simulink model "MPC_linear_2015"  (R2015a)
settings: Solver=ode45  StartTime=0.0  StopTime=10.0  RelTol=1e-3
values from neighbouring files (symbols this model uses):
  AINEQ = mpcobj.AINEQ    [teste.m]
  cmd_lb = -1e5    (= -100000)    [initParams.m]    (also in teste.m = -2000)
  cmd_ub = 1e5    (= 100000)    [initParams.m]    (also in teste.m = 2000)
  dA = d_sys.a    [teste.m]
  dB = d_sys.b    [teste.m]
  dC = d_sys.c    [teste.m]
  dD = d_sys.d    [teste.m]
  F1 = mpcobj.F1    [teste.m]
  F2 = mpcobj.F2    [teste.m]
  F3 = mpcobj.F3    [teste.m]
  G1 = mpcobj.G1    [teste.m]
  G2 = mpcobj.G2    [teste.m]
  G3 = mpcobj.G3    [teste.m]
  G4 = mpcobj.G4    [teste.m]
  H = mpcobj.H    [teste.m]
  lb = [ -pi/36; -pi; -pi; -pi/36 ]    [initParams.m]    (also in teste.m = -0.0872664625997)
  openloop = 0    [teste.m]
  PI = mpcobj.PI_E    [teste.m]
  rate_factor = 14    [teste.m]
  rate_lb = -rate_ub    (= -1.3962634016e-05)    [teste.m]
  rate_th = pi*Ts/180    (= 1.3962634016e-06)    [teste.m]
  rate_ub = 10*pi*Ts/180    (= 1.3962634016e-05)    [teste.m]
  ub = -lb    [initParams.m]    (also in teste.m = 0.0872664625997)
settings Model: Creator=zoero  LastModifiedBy=zoero

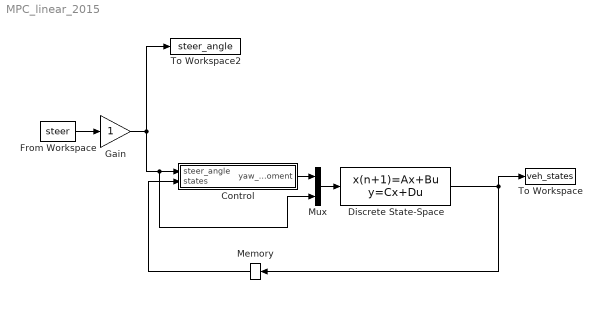
== system MPC_linear_2015 ==
  "Control " : Subsystem  TreatAsAtomicUnit=on
  Discrete State-Space : DiscreteStateSpace  A=dA  B=dB  C=dC  D=dD  X0=[0 0 0 0]  SampleTime=8e-5
  From Workspace : FromWorkspace  VariableName=steer  SampleTime=0
  Gain : Gain
  Memory : Memory  X0=[0,0,0,0]
  Mux : Mux  Inputs=2
  To Workspace : ToWorkspace  VariableName=veh_states  SaveFormat=Timeseries  SampleTime=-1
  To Workspace2 : ToWorkspace  VariableName=steer_angle  SaveFormat=Timeseries  SampleTime=-1
  wires:
  From Workspace/1 -> Gain/1
  Gain/1 -> To Workspace2/1, Mux/2, "Control "/1(steer_angle)
  Memory/1 -> "Control "/2(states)
  Discrete State-Space/1 -> To Workspace/1, Memory/1
  "Control "/1(yaw_moment) -> Mux/1
  Mux/1 -> Discrete State-Space/1

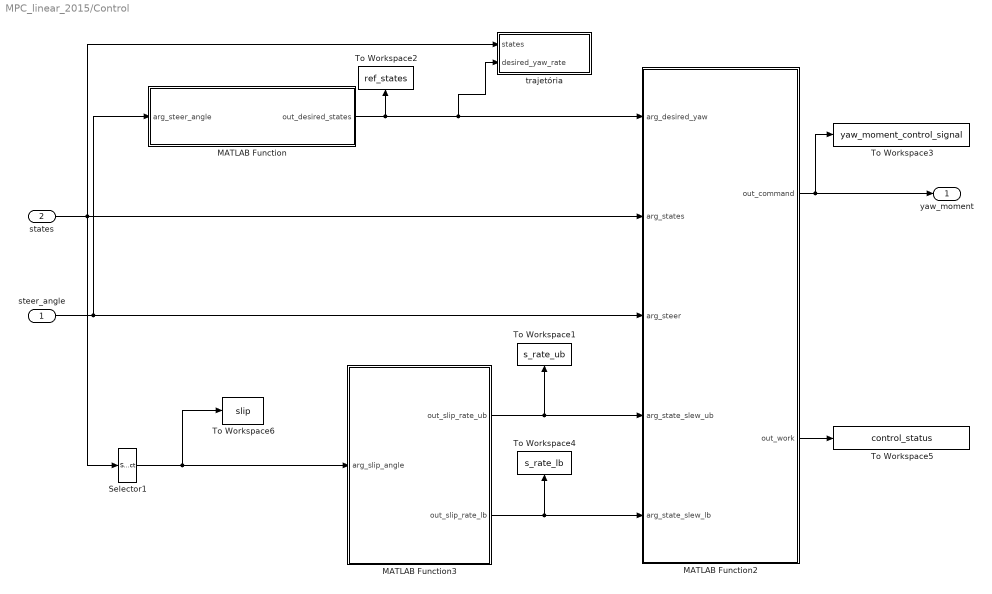
== system MPC_linear_2015/Control  ==
  steer_angle : Inport
  states : Inport  Port=2
  MATLAB Function : MATLAB Function  TreatAsAtomicUnit=on
  MATLAB Function2 : MATLAB Function  TreatAsAtomicUnit=on  SystemSampleTime=8e-5
  MATLAB Function3 : MATLAB Function  TreatAsAtomicUnit=on
  Selector1 : Selector  InputPortWidth=4  Indices=[1]
  To Workspace1 : ToWorkspace  VariableName=s_rate_ub  SaveFormat=Timeseries  SampleTime=-1
      settings: MaxDataPoints=Inf
  To Workspace2 : ToWorkspace  VariableName=ref_states  SaveFormat=Timeseries  SampleTime=-1
      settings: MaxDataPoints=Inf
  To Workspace3 : ToWorkspace  VariableName=yaw_moment_control_signal  SaveFormat=Timeseries  SampleTime=-1
      settings: MaxDataPoints=Inf
  To Workspace4 : ToWorkspace  VariableName=s_rate_lb  SaveFormat=Timeseries  SampleTime=-1
      settings: MaxDataPoints=Inf
  To Workspace5 : ToWorkspace  VariableName=control_status  SaveFormat=Timeseries  SampleTime=-1
      settings: MaxDataPoints=Inf
  To Workspace6 : ToWorkspace  VariableName=slip  SaveFormat=Timeseries  SampleTime=-1
      settings: MaxDataPoints=Inf
  trajetória : Subsystem
  yaw_moment : Outport
  wires:
  MATLAB Function2/1(out_command) -> To Workspace3/1, yaw_moment/1
  steer_angle/1 -> MATLAB Function/1(arg_steer_angle), MATLAB Function2/3(arg_steer)
  MATLAB Function3/1(out_slip_rate_ub) -> To Workspace1/1, MATLAB Function2/4(arg_state_slew_ub)
  MATLAB Function3/2(out_slip_rate_lb) -> MATLAB Function2/5(arg_state_slew_lb), To Workspace4/1
  states/1 -> MATLAB Function2/2(arg_states), Selector1/1, trajetória/1(states)
  MATLAB Function2/2(out_work) -> To Workspace5/1
  Selector1/1 -> To Workspace6/1, MATLAB Function3/1(arg_slip_angle)
  MATLAB Function/1(out_desired_states) -> To Workspace2/1, trajetória/2(desired_yaw_rate), MATLAB Function2/1(arg_desired_yaw)

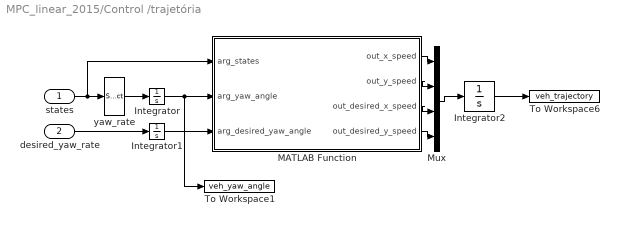
== system MPC_linear_2015/Control /trajetória ==
  states : Inport
  desired_yaw_rate : Inport  Port=2
  Integrator : Integrator
  Integrator1 : Integrator
  Integrator2 : Integrator
  MATLAB Function : MATLAB Function  TreatAsAtomicUnit=on
  Mux : Mux
  To Workspace1 : ToWorkspace  VariableName=veh_yaw_angle  SaveFormat=Timeseries  SampleTime=-1
  To Workspace6 : ToWorkspace  VariableName=veh_trajectory  SaveFormat=Timeseries  SampleTime=-1
  yaw_rate : Selector  InputPortWidth=4  Indices=[2]
  wires:
  states/1 -> yaw_rate/1, MATLAB Function/1(arg_states)
  yaw_rate/1 -> Integrator/1
  Integrator/1 -> To Workspace1/1, MATLAB Function/2(arg_yaw_angle)
  Integrator1/1 -> MATLAB Function/3(arg_desired_yaw_angle)
  desired_yaw_rate/1 -> Integrator1/1
  MATLAB Function/1(out_x_speed) -> Mux/1
  MATLAB Function/2(out_y_speed) -> Mux/2
  MATLAB Function/3(out_desired_x_speed) -> Mux/3
  MATLAB Function/4(out_desired_y_speed) -> Mux/4
  Mux/1 -> Integrator2/1
  Integrator2/1 -> To Workspace6/1

== matlab function MPC_linear_2015/Control /MATLAB Function ==
  data: arg_steer_angle input; out_desired_states output; uspeed parameter
function out_desired_states  = desired_states(arg_steer_angle,  uspeed)

persistent mu_g;
persistent Ku;
persistent l;

if isempty(Ku)
    modelParams = coder.load( 'modelParam.mat' );
    mu_g = modelParams.friction_coefficient*modelParams.g;
    l = modelParams.l;
    Ku = modelParams.Ku;
end

aux = (l + Ku*uspeed*uspeed);
desired_yaw_rate = uspeed*arg_steer_angle/aux;


desired_yaw_rate = min([abs(desired_yaw_rate), abs(mu_g/uspeed)])*sign(arg_steer_angle);


out_desired_states = desired_yaw_rate;

end

== matlab function MPC_linear_2015/Control /MATLAB Function2 ==
  data: arg_desired_yaw input; out_command output size=1; arg_states input; arg_steer input; arg_state_slew_ub input; arg_state_slew_lb input; G1 parameter; G2 parameter; G3 parameter; G4 parameter; F1 parameter; F2 parameter; F3 parameter; cmd_lb parameter; cmd_ub parameter; H parameter; AINEQ parameter; PI parameter; ub parameter; lb parameter; out_work output; openloop parameter
function [out_command, out_work]= mpc(arg_desired_yaw, arg_states, arg_steer, ...
arg_state_slew_ub, arg_state_slew_lb, G1, G2, G3, G4, F1, F2, F3, cmd_lb,...
cmd_ub, H, AINEQ, PI, ub,lb, openloop)
 persistent U
 persistent QP
 persistent N
 persistent np
 persistent nc
 persistent nu
% persistent on
 if isempty(U)
     U = 0;
     N = 101;
     np = 4;
     nc = 1;
     nu = 2;
 %    on = 0;
 end
 
 if  openloop ~= 0
    out_command = 0;
    out_work = 0;
    return
 end
  %if on == 0
  %  if ( abs(arg_desired_yaw) > pi/180) || ( abs(arg_states(1)) > 4*pi/180 )
  %      on = 1;
  %  else
  %      out_command = 0;
  %      return;
  %  end
  %else
  %  if ( abs(arg_desired_yaw) < pi/180 ) && ( abs(arg_states(1)) < 4*pi/180 )
  %      out_command = 0;
  %      %on = 0;
  %      %return;
  %  end
  %end
 
 TRACK = arg_desired_yaw*ones(N,1);
 TRACK = reshape(TRACK,[],1);
 G5 = zeros(8*N,1);
 G5( 6*N+1:7*N, : ) = repmat(arg_state_slew_ub,N,1);
 G5( 7*N+1:8*N, : ) = -repmat(arg_state_slew_lb,N,1);
 
 B_INEQ = ( G1 + G4 )*arg_states + G2*U + G3 + G5;
 F = F1*arg_states + F2*TRACK + F3*[0; arg_steer];
 F = PI'*F;
 aux_cmd_lb = repmat([cmd_lb;arg_steer],N,1);    
 aux_cmd_ub = repmat([cmd_ub;arg_steer],N,1);
 B_INEQ = [B_INEQ(1:606,:);-aux_cmd_lb;aux_cmd_ub];
 
 exitflag = 0;

 coder.extrinsic('qpOASES_sequence'); 
 
    if isempty(QP)
        [QP,p,fval,exitflag,iter] = qpOASES_sequence( 'i', H,F,AINEQ([1:606,809:end],:),[ ones(np-1,1)*aux_cmd_lb(1); aux_cmd_lb(2)],[ ones(np-1,1)*aux_cmd_ub(1); aux_cmd_ub(2)],[], B_INEQ, 2000 );
    else
        [p,fval,exitflag,iter] = qpOASES_sequence( 'h', QP,F,[ ones(np-1,1)*aux_cmd_lb(1); aux_cmd_lb(2)],[ ones(np-1,1)*aux_cmd_ub(1); aux_cmd_ub(2)],[], B_INEQ, 100 );
    end
    
    if exitflag == (-2)
        %Correcao de erro numero da otimizacao quando o estado restrito tem
        %Condicao inicial fora da restricao.
        %O que esta sendo feito aqui e definir um perfil de restricao
        %igual a um decaimento exponencial do valor atual para
        %um valor dentro da restricao.
        if arg_states(1) > ub
            bound = 2* ub -  arg_states(1) + 2*(arg_states(1) - ub)* exp(-(0:N-1)/20) ;
            newG3 = G3;
            newG3(1:N*nc,1) = bound';
        elseif arg_states(1) < lb
            bound = 2*lb  -  arg_states(1) + 2*(arg_states(1) - lb)* exp(-(0:N-1)/20) ;
            newG3 = G3;
            newG3(N*nc+1:2*N*nc,1) = -bound';
        else
            out_command = U;
            out_work = 1000;
            return;
        end
            
        B_INEQ = ( G1 + G4)*arg_states + G2*U + newG3 + G5;
        B_INEQ = [B_INEQ(1:606,:);-aux_cmd_lb;aux_cmd_ub];

        exitflag = 0;
        [p,fval,exitflag,iter] = qpOASES_sequence( 'h', QP,F,[ ones(np-1,1)*aux_cmd_lb(1); aux_cmd_lb(2)],[ ones(np-1,1)*aux_cmd_ub(1); aux_cmd_ub(2)],[], B_INEQ, 100 ); 
        if exitflag == (-2)
            out_command = U;
            out_work = 1000;
        else
            out_work = -1000;
            out_command = PI(1,:)*p;
        end
    else
        out_work = 0;
        out_command = PI(1,:)*p;
    end
    
    U = out_command;
end

== matlab function MPC_linear_2015/Control /MATLAB Function3 ==
  data: arg_slip_angle input; out_slip_rate_ub output; out_slip_rate_lb output; rate_lb parameter; rate_ub parameter; lb parameter; ub parameter; rate_factor parameter; rate_th parameter
function [out_slip_rate_ub,out_slip_rate_lb] = fcn(arg_slip_angle, rate_lb, rate_ub, lb, ub, rate_factor, rate_th)

    out_slip_rate_ub = atan((( ub - arg_slip_angle )/(ub - lb))*rate_factor)*rate_ub;
    out_slip_rate_lb = atan((( arg_slip_angle - lb )/(ub - lb))*rate_factor)*rate_lb;
    out_slip_rate_ub( out_slip_rate_ub < rate_th ) = rate_th;
    out_slip_rate_lb( out_slip_rate_lb > -rate_th ) = -rate_th;
end

== matlab function MPC_linear_2015/Control /trajetória/MATLAB Function ==
  data: arg_states input; out_x_speed output; arg_yaw_angle input; arg_desired_yaw_angle input; out_y_speed output; out_desired_x_speed output; out_desired_y_speed output
function [out_x_speed, out_y_speed, out_desired_x_speed, out_desired_y_speed] = speed( arg_states, arg_yaw_angle, arg_desired_yaw_angle )

out_x_speed = arg_states(2)*cos(arg_yaw_angle) - arg_states(1)*sin(arg_yaw_angle);
out_y_speed = arg_states(2)*sin(arg_yaw_angle) + arg_states(1)*cos(arg_yaw_angle);
out_desired_x_speed = arg_states(2)*cos(arg_desired_yaw_angle) - arg_states(1)*sin(arg_desired_yaw_angle);
out_desired_y_speed = arg_states(2)*sin(arg_desired_yaw_angle) + arg_states(1)*cos(arg_desired_yaw_angle);


end
